simulink model "LBSSHA005_EEE4119F_Project"  (R2021a)
settings: Solver=VariableStepAuto  StartTime=0.0  StopTime=60  RelTol=1e-3
undefined symbols (not defined in the file or in its folder): Klqr, Klqr_b, Kr, Kr_b
libraries: dspsigops x1
settings Model: EnablePacing=on  Creator=Administrator  LastModifiedBy=shaun
settings SolverCC: ZeroCrossAlgorithm=Adaptive
settings DebuggingCC: IgnoredZcDiagnostic=none

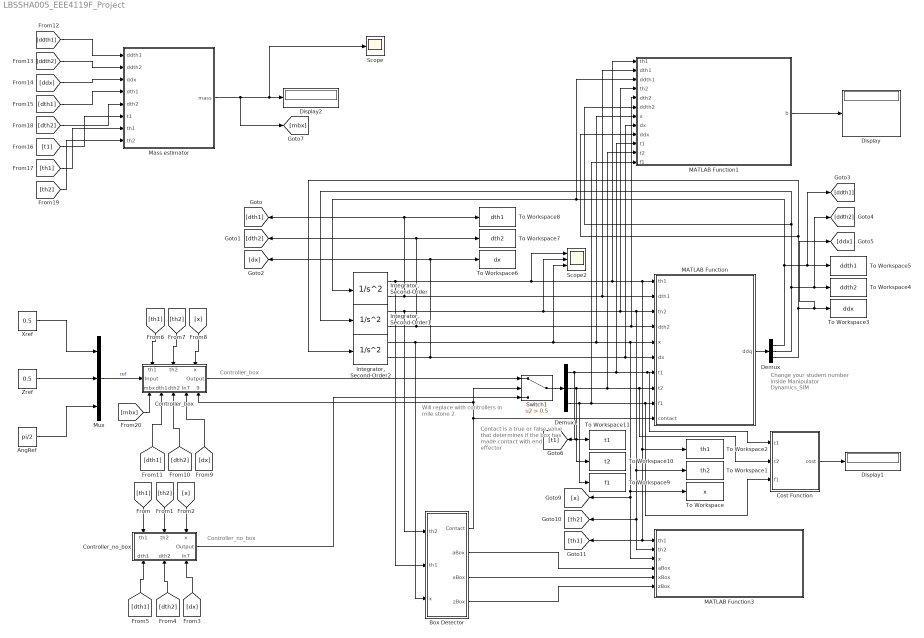
== system LBSSHA005_EEE4119F_Project ==
  note: Controller_box
  note: Controller_no_box
  note: Contact is a true or false value that determines if the box has made contact with end effector
  note: Will replace with controllers in mile stone 2
  note: Change your student number inside Manipulator Dynamics_SIM
  AngRef : Constant  Value=pi/2
  Box Detector : Subsystem
  Controller_box : Subsystem
      settings: PortSchema="{\"entries\":[{\"content\":{\"sides\":[{\"content\":{\"connectorIds\":[\"In1\"]},\"type\":\"ConnectorPlacement.EquallySpacedRectSide\",\"uuid\":\"442c6cb1-0c83-47f7-ad07-2f020ac45e6e\"},{\"content\":{\"connectorIds\":[\"Out1\"],\"side\":\"RIGHT\"},\"type\":\"ConnectorPlacement.EquallySpacedRectSide\",\"uuid\":\"7f993a2f-adf1-4607-9f11-cdbb59b13442\"},{\"content\":{\"connectorIds\":[\"In2\",\"In3\",\"In4\"],\"side\":\"TOP\"},\"type\":\"ConnectorPlacement.EquallySpacedRectSide\",\"uuid\":\"5e67f2e7-af9c-4bde-80a5-b1ef30d10dbb\"},{\"content\":{\"connectorIds\":[\"In5\",\"In6\",\"In7\",\"In8\",\"In9\"],\"side\":\"BOTTOM\"},\"type\":\"ConnectorPlacement.EquallySpacedRectSide\",\"uuid\":\"20da8873-f5b9-43e3-93ec-958325ed584f\"}]},\"type\":\"ConnectorPlacement.EquallySpacedConnector\",\"uuid\":\"88c068a2-7487-43c4-b188-48c79a1dd5d7\"}],\"packageUris\":[\"http://schema.mathworks.com/mf0/Connector/R2020b\"],\"version\":\"1.0\"}"
  Controller_no_box : Subsystem
      settings: PortSchema="{\"entries\":[{\"content\":{\"sides\":[{\"content\":{\"connectorIds\":[]},\"type\":\"ConnectorPlacement.EquallySpacedRectSide\",\"uuid\":\"88738e74-d91b-4dc7-a725-58f175a94349\"},{\"content\":{\"connectorIds\":[\"Out1\"],\"side\":\"RIGHT\"},\"type\":\"ConnectorPlacement.EquallySpacedRectSide\",\"uuid\":\"6cf3a578-d327-404a-bf63-fc00ab4a30ba\"},{\"content\":{\"connectorIds\":[\"In1\",\"In2\",\"In3\"],\"side\":\"TOP\"},\"type\":\"ConnectorPlacement.EquallySpacedRectSide\",\"uuid\":\"b92cd528-6e23-44bd-9603-b71daa2ffdae\"},{\"content\":{\"connectorIds\":[\"In4\",\"In5\",\"In6\"],\"side\":\"BOTTOM\"},\"type\":\"ConnectorPlacement.EquallySpacedRectSide\",\"uuid\":\"f1bd1ac8-fd96-4684-af34-69bf2dd321d9\"}]},\"type\":\"ConnectorPlacement.EquallySpacedConnector\",\"uuid\":\"af1ac5a9-5139-4c84-9774-81cc3394ecc5\"}],\"packageUris\":[\"http://schema.mathworks.com/mf0/Connector/R2020b\"],\"version\":\"1.0\"}"
  Cost Function : Subsystem
  Demux : Demux  Outputs=3
  Demux1 : Demux  Outputs=3
  Display : Display
  Display1 : Display
  Display2 : Display
  "Integrator, Second-Order" : SecondOrderIntegrator
  "Integrator, Second-Order1" : SecondOrderIntegrator  ICX=0
  "Integrator, Second-Order2" : SecondOrderIntegrator  ICX=0
  MATLAB Function : MATLAB Function  TreatAsAtomicUnit=on
  MATLAB Function1 : MATLAB Function  TreatAsAtomicUnit=on
  MATLAB Function3 : MATLAB Function  TreatAsAtomicUnit=on  SystemSampleTime=0.15
  Mass estimator : MATLAB Function  TreatAsAtomicUnit=on
  Mux : Mux  Inputs=3
  Scope : Scope
  Scope2 : Scope  NumInputPorts=3
  Switch1 : Switch  Criteria=u2 > Threshold  Threshold=0.5
  To Workspace : ToWorkspace  VariableName=x  SaveFormat=Structure With Time  SampleTime=-1
  To Workspace1 : ToWorkspace  VariableName=th2  SaveFormat=Structure With Time  SampleTime=-1
  To Workspace10 : ToWorkspace  VariableName=t2  SaveFormat=Structure With Time  SampleTime=-1
  To Workspace11 : ToWorkspace  VariableName=t1  SaveFormat=Structure With Time  SampleTime=-1
  To Workspace2 : ToWorkspace  VariableName=th1  SaveFormat=Structure With Time  SampleTime=-1
  To Workspace3 : ToWorkspace  VariableName=ddx  SaveFormat=Structure With Time  SampleTime=-1
  To Workspace4 : ToWorkspace  VariableName=ddth2  SaveFormat=Structure With Time  SampleTime=-1
  To Workspace5 : ToWorkspace  VariableName=ddth1  SaveFormat=Structure With Time  SampleTime=-1
  To Workspace6 : ToWorkspace  VariableName=dx  SaveFormat=Structure With Time  SampleTime=-1
  To Workspace7 : ToWorkspace  VariableName=dth2  SaveFormat=Structure With Time  SampleTime=-1
  To Workspace8 : ToWorkspace  VariableName=dth1  SaveFormat=Structure With Time  SampleTime=-1
  To Workspace9 : ToWorkspace  VariableName=f1  SaveFormat=Structure With Time  SampleTime=-1
  Xref : Constant  Value=0.5
  Zref : Constant  Value=0.5
  wires:
  Demux/1 -> [ddth1], To Workspace5/1, MATLAB Function1/3(ddth1), "Integrator, Second-Order"/1
  Demux/2 -> [ddth2], To Workspace4/1, MATLAB Function1/6(ddth2), "Integrator, Second-Order1"/1
  MATLAB Function/1(ddq) -> Demux/1
  "Integrator, Second-Order1"/2 -> [dth2], To Workspace7/1, MATLAB Function1/5(dth2), MATLAB Function/4(dth2)
  Demux1/1 -> [t1], To Workspace11/1, MATLAB Function1/10(t1), Cost Function/1(t1), MATLAB Function/7(t1)
  "Integrator, Second-Order"/1 -> Box Detector/2(th1), Scope2/1, MATLAB Function1/1(th1), MATLAB Function3/1(th1), [th1], To Workspace2/1, MATLAB Function/1(th1)
  "Integrator, Second-Order1"/1 -> Box Detector/1(th2), [th2], MATLAB Function3/2(th2), To Workspace1/1, MATLAB Function/3(th2), MATLAB Function1/4(th2), Scope2/2
  "Integrator, Second-Order2"/2 -> [dx], To Workspace6/1, MATLAB Function1/8(dx), MATLAB Function/6(dx)
  Demux/3 -> [ddx], To Workspace3/1, MATLAB Function1/9(ddx), "Integrator, Second-Order2"/1
  "Integrator, Second-Order2"/1 -> Scope2/3, MATLAB Function1/7(x), [x], MATLAB Function3/3(x), To Workspace/1, MATLAB Function/5(x), Box Detector/3(x)
  "Integrator, Second-Order"/2 -> To Workspace8/1, [dth1], MATLAB Function1/2(dth1), MATLAB Function/2(dth1)
  Demux1/2 -> To Workspace10/1, Cost Function/2(t2), MATLAB Function/8(t2), MATLAB Function1/11(t2)
  Demux1/3 -> To Workspace9/1, Cost Function/3(f1), MATLAB Function/9(f1), MATLAB Function1/12(f1)
  Switch1/1 -> Demux1/1
  Box Detector/4(zBox) -> MATLAB Function3/6(zBox)
  Box Detector/3(xBox) -> MATLAB Function3/5(xBox)
  Box Detector/2(aBox) -> MATLAB Function3/4(aBox)
  Box Detector/1(Contact) -> Controller_box/9(Contact), Switch1/2, MATLAB Function/10(contact)
  MATLAB Function1/1(b) -> Display/1
  [th1] -> Controller_no_box/1(th1)
  [th2] -> Controller_no_box/2(th2)
  [x] -> Controller_no_box/3(x)
  [dth1] -> Controller_no_box/4(dth1)
  [dth2] -> Controller_no_box/5(dth2)
  [dx] -> Controller_no_box/6(In7)
  [th2] -> Controller_box/3(th2)
  [th1] -> Controller_box/2(th1)
  [x] -> Controller_box/4(x)
  [dx] -> Controller_box/8(In7)
  [dth2] -> Controller_box/7(dth2)
  [dth1] -> Controller_box/6(dth1)
  Controller_box/1(Output) -> Switch1/1
  Controller_no_box/1(Output) -> Switch1/3
  Zref/1 -> Mux/2
  Xref/1 -> Mux/1
  AngRef/1 -> Mux/3
  Mux/1 -> Controller_box/1(Input)  "ref"
  Cost Function/1(cost) -> Display1/1
  [ddth1] -> Mass estimator/1(ddth1)
  [ddth2] -> Mass estimator/2(ddth2)
  [ddx] -> Mass estimator/3(ddx)
  [dth1] -> Mass estimator/4(dth1)
  [dth2] -> Mass estimator/5(dth2)
  [t1] -> Mass estimator/6(t1)
  [th1] -> Mass estimator/7(th1)
  [th2] -> Mass estimator/8(th2)
  Mass estimator/1(mass) -> [mbx], Scope/1, Display2/1
  [mbx] -> Controller_box/5(mbx)

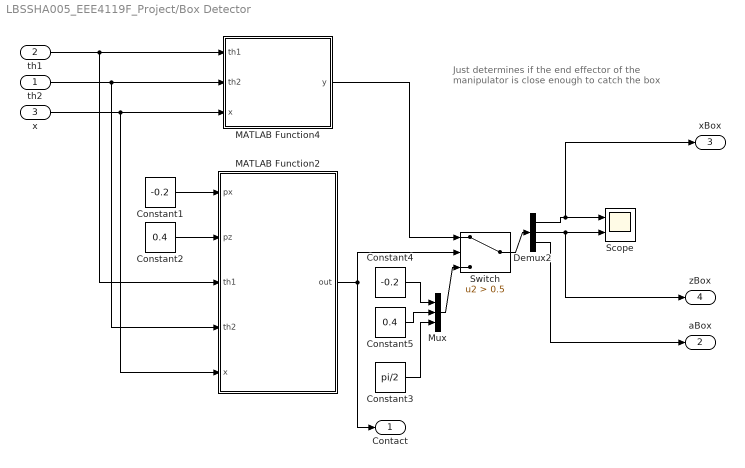
== system LBSSHA005_EEE4119F_Project/Box Detector ==
  note: Just determines if the end effector of the manipulator is close enough to catch the box
  th2 : Inport
  th1 : Inport  Port=2
  x : Inport  Port=3
  Constant1 : Constant  Value=-0.2
  Constant2 : Constant  Value=0.4
  Constant3 : Constant  Value=pi/2
  Constant4 : Constant  Value=-0.2
  Constant5 : Constant  Value=0.4
  Demux2 : Demux  Outputs=3
  MATLAB Function2 : MATLAB Function  TreatAsAtomicUnit=on
  MATLAB Function4 : MATLAB Function  TreatAsAtomicUnit=on
  Mux : Mux  Inputs=3
  Scope : Scope  NumInputPorts=2
  Switch : Switch  Criteria=u2 > Threshold  Threshold=0.5
  Contact : Outport
  aBox : Outport  Port=2
  xBox : Outport  Port=3
  zBox : Outport  Port=4
  wires:
  Demux2/2 -> zBox/1, Scope/2
  Mux/1 -> Switch/3
  Constant5/1 -> Mux/2
  MATLAB Function4/1(y) -> Switch/1
  Demux2/1 -> Scope/1, xBox/1
  Constant4/1 -> Mux/1
  Switch/1 -> Demux2/1
  x/1 -> MATLAB Function2/5(x), MATLAB Function4/3(x)
  th1/1 -> MATLAB Function2/3(th1), MATLAB Function4/1(th1)
  th2/1 -> MATLAB Function2/4(th2), MATLAB Function4/2(th2)
  MATLAB Function2/1(out) -> Switch/2, Contact/1
  Constant1/1 -> MATLAB Function2/1(px)
  Constant2/1 -> MATLAB Function2/2(pz)
  Demux2/3 -> aBox/1
  Constant3/1 -> Mux/3

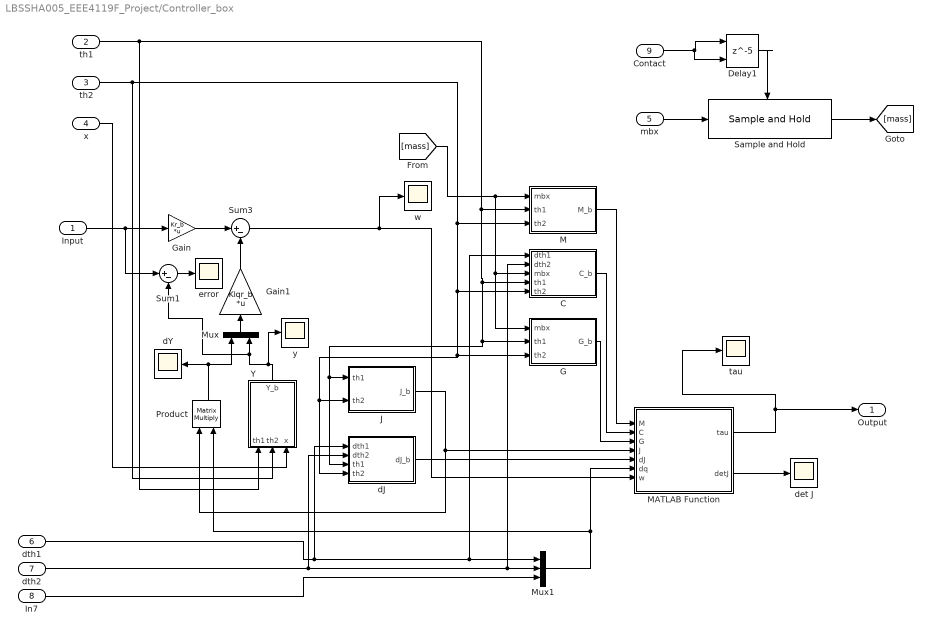
== system LBSSHA005_EEE4119F_Project/Controller_box ==
  Input : Inport
  th1 : Inport  Port=2
  th2 : Inport  Port=3
  x : Inport  Port=4
  mbx : Inport  Port=5
  dth1 : Inport  Port=6
  dth2 : Inport  Port=7
  In7 : Inport  Port=8
  Contact : Inport  Port=9
  C : MATLAB Function  TreatAsAtomicUnit=on
  Delay1 : Delay  DelayLength=5  ExternalReset=Rising
      settings: InputPortMap=u0,r5
  G : MATLAB Function  TreatAsAtomicUnit=on
  Gain : Gain  Gain=Kr_b  Multiplication=Matrix(K*u)
  Gain1 : Gain  Gain=Klqr_b  Multiplication=Matrix(K*u)
  J : MATLAB Function  TreatAsAtomicUnit=on
  M : MATLAB Function  TreatAsAtomicUnit=on
  MATLAB Function : MATLAB Function  TreatAsAtomicUnit=on
  Mux : Mux  Inputs=2
  Mux1 : Mux  Inputs=3
  Product : Product  Multiplication=Matrix(*)
  Sample and Hold : dspsigops/Sample and Hold  trig=Rising edge  initCond=1  latchinput=on
  Sum1 : Sum  Inputs=|+-
  Sum3 : Sum  Inputs=|+-
  Y : MATLAB Function  TreatAsAtomicUnit=on
  dJ : MATLAB Function  TreatAsAtomicUnit=on
  dY : Scope
  det J : Scope
  error : Scope
  tau : Scope
  w : Scope
  y : Scope
  Output : Outport
  wires:
  J/1(J_b) -> MATLAB Function/4(J), Product/1
  Gain1/1 -> Sum3/2
  Y/1(Y_b) -> Sum1/2, Mux/2, y/1
  Product/1 -> dY/1, Mux/1
  MATLAB Function/1(tau) -> Output/1, tau/1
  Mux/1 -> Gain1/1
  dJ/1(dJ_b) -> MATLAB Function/5(dJ)
  Sum3/1 -> MATLAB Function/7(w), w/1
  Input/1 -> Gain/1, Sum1/1
  MATLAB Function/2(detJ) -> det J/1
  Sum1/1 -> error/1
  M/1(M_b) -> MATLAB Function/1(M)
  C/1(C_b) -> MATLAB Function/2(C)
  G/1(G_b) -> MATLAB Function/3(G)
  th1/1 -> Y/1(th1), G/2(th1), dJ/3(th1), J/1(th1), C/4(th1), M/2(th1)
  th2/1 -> Y/2(th2), G/3(th2), dJ/4(th2), J/2(th2), C/5(th2), M/3(th2)
  x/1 -> Y/3(x)
  dth1/1 -> C/1(dth1), Mux1/1, dJ/1(dth1)
  dth2/1 -> C/2(dth2), Mux1/2, dJ/2(dth2)
  In7/1 -> Mux1/3
  Mux1/1 -> MATLAB Function/6(dq), Product/2
  Gain/1 -> Sum3/1
  Delay1/1 -> Sample and Hold/Trigger
  Sample and Hold/1 -> [mass]
  [mass] -> M/1(mbx), G/1(mbx), C/3(mbx)
  mbx/1 -> Sample and Hold/1
  Contact/1 -> Delay1/2, Delay1/1

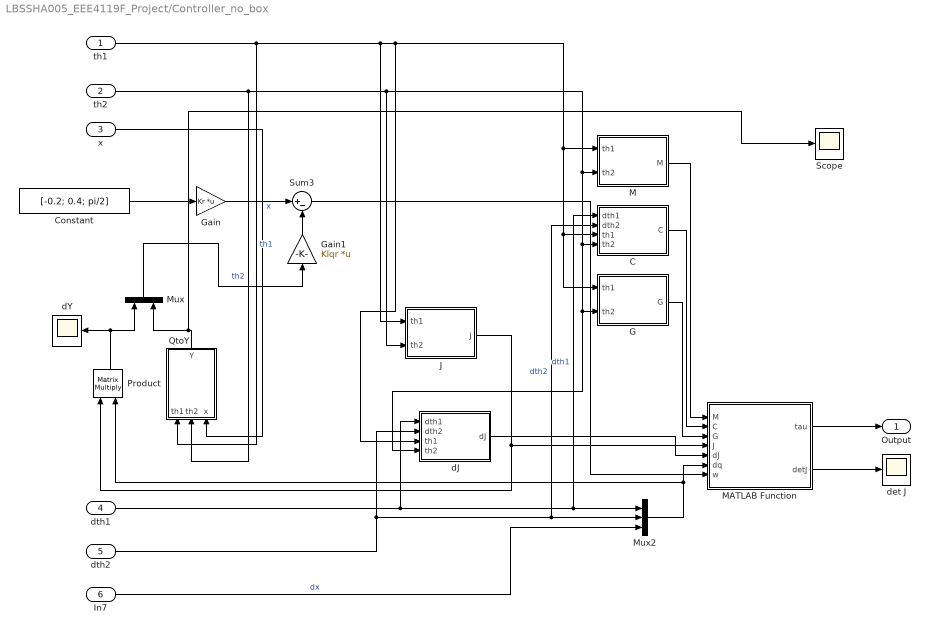
== system LBSSHA005_EEE4119F_Project/Controller_no_box ==
  th1 : Inport
  th2 : Inport  Port=2
  x : Inport  Port=3
  dth1 : Inport  Port=4
  dth2 : Inport  Port=5
  In7 : Inport  Port=6
  C : MATLAB Function  TreatAsAtomicUnit=on
  Constant : Constant  Value=[-0.2; 0.4; pi/2]
  G : MATLAB Function  TreatAsAtomicUnit=on
  Gain : Gain  Gain=Kr  Multiplication=Matrix(K*u)
  Gain1 : Gain  Gain=Klqr  Multiplication=Matrix(K*u)
  J : MATLAB Function  TreatAsAtomicUnit=on
  M : MATLAB Function  TreatAsAtomicUnit=on
  MATLAB Function : MATLAB Function  TreatAsAtomicUnit=on
  Mux : Mux  Inputs=2
  Mux2 : Mux  Inputs=3
  Product : Product  Multiplication=Matrix(*)
  QtoY : MATLAB Function  TreatAsAtomicUnit=on
  Scope : Scope
  Sum3 : Sum  Inputs=|+-
  dJ : MATLAB Function  TreatAsAtomicUnit=on
  dY : Scope
  det J : Scope
  Output : Outport
  wires:
  M/1(M) -> MATLAB Function/1(M)
  J/1(J) -> MATLAB Function/4(J), Product/1
  Gain1/1 -> Sum3/2
  QtoY/1(Y) -> Scope/1, Mux/2
  Product/1 -> dY/1, Mux/1
  MATLAB Function/1(tau) -> Output/1
  Mux/1 -> Gain1/1
  dJ/1(dJ) -> MATLAB Function/5(dJ)
  Sum3/1 -> MATLAB Function/7(w)
  Constant/1 -> Gain/1
  C/1(C) -> MATLAB Function/2(C)
  MATLAB Function/2(detJ) -> det J/1
  dth1/1 -> C/1(dth1), Mux2/1, dJ/1(dth1)  "dth1"
  dth2/1 -> C/2(dth2), Mux2/2, dJ/2(dth2)  "dth2"
  In7/1 -> Mux2/3  "dx"
  Mux2/1 -> MATLAB Function/6(dq), Product/2
  th2/1 -> J/2(th2), C/4(th2), dJ/4(th2), G/2(th2), M/2(th2), QtoY/2(th2)  "th2"
  x/1 -> QtoY/3(x)  "x"
  th1/1 -> dJ/3(th1), C/3(th1), G/1(th1), M/1(th1), J/1(th1), QtoY/1(th1)  "th1"
  G/1(G) -> MATLAB Function/3(G)
  Gain/1 -> Sum3/1

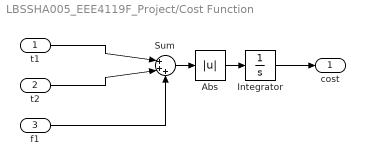
== system LBSSHA005_EEE4119F_Project/Cost Function ==
  t1 : Inport
  t2 : Inport  Port=2
  f1 : Inport  Port=3
  Abs : Abs
  Integrator : Integrator
  Sum : Sum  Inputs=|+++
  cost : Outport
  wires:
  Sum/1 -> Abs/1
  f1/1 -> Sum/3
  t2/1 -> Sum/2
  Integrator/1 -> cost/1
  t1/1 -> Sum/1
  Abs/1 -> Integrator/1

== matlab function LBSSHA005_EEE4119F_Project/Controller_no_box/C ==
  data: C output; dth1 input; dth2 input; th1 input; th2 input
function C = C(dth1,dth2,th1,th2)
%#codegen

%    This function was generated by the Symbolic Math Toolbox version 8.7.
%    13-May-2022 16:47:02

t2 = sin(th2);
t3 = th1+th2;
t4 = cos(t3);
C = [dth2.*t2.*(dth1.*2.0+dth2).*(-1.0./1.28e+2);(dth1.^2.*t2)./1.28e+2;-dth1.*(dth1.*(t4./3.2e+1+cos(th1).*(3.0./3.2e+1))+(dth2.*t4)./3.2e+1)-(dth2.*t4.*(dth1+dth2))./3.2e+1];

== matlab function LBSSHA005_EEE4119F_Project/Controller_no_box/QtoY ==
  data: th1 input; Y output; th2 input; x input
function Y = QtoY(th1,th2,x)
%#codegen

%    This function was generated by the Symbolic Math Toolbox version 8.7.
%    13-May-2022 16:47:02

t2 = cos(th1);
t3 = cos(th2);
t4 = sin(th1);
t5 = sin(th2);
Y = [t2./4.0+x+(t2.*t3)./4.0-(t4.*t5)./4.0;t4./4.0+(t2.*t5)./4.0+(t3.*t4)./4.0;th1+th2];

== matlab function LBSSHA005_EEE4119F_Project/Controller_box/MATLAB Function ==
  data: M input; tau output; C input; G input; J input; dJ input; dq input; w input; detJ output
function [tau,detJ] = fcn(M, C, G, J, dJ, dq, w)

% Mapping the nonlinear control - used Jacobian Transpose Method
% (https://journals.sagepub.com/doi/pdf/10.1177/0278364917698748)
% J\ - could try this...
% pinv(J) - could also try this...
% Check that Jaocbian is not singular. If singular rather use transpose.
b = 0.8353;
G = transpose(G);
if abs(det(J)) < 1e-3
    tau = M*(J'*(w-dJ*dq)) + C + G + b*dq;
else
    tau = M*(J\(w-dJ*dq)) + C + G + b*dq;
end

detJ = det(J);
% see http://www.cs.columbia.edu/~allen/F15/NOTES/jacobians.pdf for further
% clarity on Jacobians going singular. Short answer: this happens when a robot loses a degree
% of freedom, similar to what we discussed in class about Gimbal Lock

== matlab function LBSSHA005_EEE4119F_Project/Controller_no_box/dJ ==
  data: dth1 input; dJ output; dth2 input; th1 input; th2 input
function dJ = dJ(dth1,dth2,th1,th2)
%#codegen

%    This function was generated by the Symbolic Math Toolbox version 8.7.
%    13-May-2022 16:47:03

t2 = th1+th2;
t3 = cos(t2);
t4 = sin(t2);
t5 = (dth2.*t3)./4.0;
t6 = (dth2.*t4)./4.0;
t7 = -t5;
t8 = -t6;
dJ = reshape([t7-(dth1.*(t3+cos(th1)))./4.0,t8-(dth1.*(t4+sin(th1)))./4.0,0.0,t7-(dth1.*t3)./4.0,t8-(dth1.*t4)./4.0,0.0,0.0,0.0,0.0],[3,3]);

== matlab function LBSSHA005_EEE4119F_Project/Controller_box/M ==
  data: mbx input; th1 input; M_b output; th2 input
function M_b = M(mbx,th1,th2)
%#codegen

%    This function was generated by the Symbolic Math Toolbox version 8.7.
%    13-May-2022 16:47:03

t2 = cos(th1);
t3 = sin(th1);
t4 = th1+th2;
t13 = mbx./3.0e+2;
t5 = cos(t4);
t6 = sin(t4);
t9 = t2./4.0;
t10 = t3./2.0;
t11 = t3./4.0;
t12 = t3.*(3.0./3.2e+1);
t7 = t5.^2;
t8 = t6.^2;
t14 = t6.*(3.0./5.0);
t15 = -t12;
t16 = t5./8.0;
t17 = t5.*(3.0./1.0e+1);
t18 = t6./8.0;
t19 = t6.*(3.0./1.0e+1);
t20 = t6./3.2e+1;
t23 = mbx.*t6.*(-3.0./1.0e+1);
t21 = -t20;
t22 = mbx.*t19;
t24 = t10+t14;
t25 = t9+t16;
t26 = t9+t17;
t27 = t11+t18;
t28 = t11+t19;
t29 = (mbx.*t24)./2.0;
t31 = t21+t23;
t32 = (t5.*t25)./3.2e+1;
t33 = t20.*t27;
t34 = mbx.*t17.*t26;
t35 = t22.*t28;
t30 = -t29;
t37 = t13+t32+t33+t34+t35+1.0./1.92e+2;
t36 = t15+t21+t30;
M_b = reshape([t13+cos(th1.*2.0)./5.12e+2+mbx.*t26.^2+mbx.*t28.^2+t3.^2./2.56e+2+t25.^2./4.0+t27.^2./4.0+1.236979166666667e-2,t37,t36,t37,t7./2.56e+2+t8./2.56e+2+t13+mbx.*t7.*(9.0./1.0e+2)+mbx.*t8.*(9.0./1.0e+2)+1.0./1.92e+2,t31,t36,t31,mbx+3.0./4.0],[3,3]);

== matlab function LBSSHA005_EEE4119F_Project/Controller_box/G ==
  data: mbx input; th1 input; G_b output; th2 input
function G_b = G(mbx,th1,th2)
%#codegen

%    This function was generated by the Symbolic Math Toolbox version 8.7.
%    13-May-2022 16:47:04

t2 = cos(th1);
t3 = th1+th2;
t4 = cos(t3);
G_b = [t2.*9.196875e-1+t4.*3.065625e-1+mbx.*(t2./4.0+t4.*(3.0./1.0e+1)).*(9.81e+2./1.0e+2),t4.*(mbx.*(3.0./5.0)+1.0./1.6e+1).*(9.81e+2./2.0e+2),0.0];

== matlab function LBSSHA005_EEE4119F_Project/Controller_box/C ==
  data: dth1 input; C_b output; dth2 input; mbx input; th1 input; th2 input
function C_b = C(dth1,dth2,mbx,th1,th2)
%#codegen

%    This function was generated by the Symbolic Math Toolbox version 8.7.
%    13-May-2022 16:47:04

t2 = cos(th1);
t3 = sin(th2);
t4 = th1+th2;
t6 = mbx.*(3.0./5.0);
t5 = cos(t4);
t8 = t6+1.0./1.6e+1;
t7 = t5./3.2e+1;
C_b = [dth2.*t3.*t8.*(dth1.*2.0+dth2).*(-1.0./8.0);(dth1.^2.*t3.*t8)./8.0;-dth1.*(dth1.*(t2.*(3.0./3.2e+1)+t7+(mbx.*(t2./2.0+t5.*(3.0./5.0)))./2.0)+dth2.*(t7+mbx.*t5.*(3.0./1.0e+1)))-(dth2.*t5.*t8.*(dth1+dth2))./2.0];

== matlab function LBSSHA005_EEE4119F_Project/Controller_box/J ==
  data: th1 input; J_b output; th2 input
function J_b = J(th1,th2)
%#codegen

%    This function was generated by the Symbolic Math Toolbox version 8.7.
%    13-May-2022 16:47:05

t2 = th1+th2;
t3 = cos(t2);
t4 = sin(t2);
t5 = t3.*(3.0./1.0e+1);
t6 = t4.*(3.0./1.0e+1);
t7 = -t6;
J_b = reshape([t7-sin(th1)./4.0,t5+cos(th1)./4.0,1.0,t7,t5,1.0,1.0,0.0,0.0],[3,3]);

== matlab function LBSSHA005_EEE4119F_Project/MATLAB Function1 ==
  data: th1 input; b output; dth1 input; ddth1 input; th2 input; dth2 input; ddth2 input; x input; dx input; ddx input; t1 input; t2 input; f1 input
function b = extractb(th1, dth1, ddth1,th2, dth2, ddth2, x, dx, ddx,t1, t2, f1)

m = 0.25;
L = 0.25;
g = 9.81;
Jyy = (1/3)*m*L^2;
dq = [dth1;dth2;dx];
t = [t1;t2;f1];
ddq = [ddth1;ddth2;ddx];

M = [2*Jyy + (3*L^2*m)/2 + L^2*m*cos(th2), Jyy + (L^2*m)/4 + (L^2*m*cos(th2))/2, - (3*L*m*sin(th1))/2 - (L*m*sin(th1 + th2))/2; Jyy + (L^2*m)/4 + (L^2*m*cos(th2))/2, (m*L^2)/4 + Jyy, -(L*m*sin(th1 + th2))/2; - (3*L*m*sin(th1))/2 - (L*m*sin(th1 + th2))/2, -(L*m*sin(th1 + th2))/2, 3*m];

G = [(L*g*m*(cos(th1 + th2) + 3*cos(th1)))/2, (L*g*m*cos(th1 + th2))/2, 0];

C = [-(L^2*dth2*m*sin(th2)*(2*dth1 + dth2))/2; (L^2*dth1^2*m*sin(th2))/2; - dth1*(dth1*((L*m*cos(th1 + th2))/2 + (3*L*m*cos(th1))/2) + (L*dth2*m*cos(th1 + th2))/2) - (L*dth2*m*cos(th1 + th2)*(dth1 + dth2))/2];

A = diag(dq);
B = -(M*ddq + C + transpose(G) - t);
b = A\B;

== matlab function LBSSHA005_EEE4119F_Project/Controller_box/dJ ==
  data: dth1 input; dJ_b output; dth2 input; th1 input; th2 input
function dJ_b = dJ(dth1,dth2,th1,th2)
%#codegen

%    This function was generated by the Symbolic Math Toolbox version 8.7.
%    13-May-2022 16:47:05

t2 = th1+th2;
t3 = cos(t2);
t4 = sin(t2);
t5 = dth2.*t3.*(3.0./1.0e+1);
t6 = dth2.*t4.*(3.0./1.0e+1);
t7 = -t5;
t8 = -t6;
dJ_b = reshape([t7-dth1.*(t3.*(3.0./1.0e+1)+cos(th1)./4.0),t8-dth1.*(t4.*(3.0./1.0e+1)+sin(th1)./4.0),0.0,t7-dth1.*t3.*(3.0./1.0e+1),t8-dth1.*t4.*(3.0./1.0e+1),0.0,0.0,0.0,0.0],[3,3]);

== matlab function LBSSHA005_EEE4119F_Project/Controller_box/Y ==
  data: th1 input; Y_b output; th2 input; x input
function Y_b = Y(th1,th2,x)
%#codegen

%    This function was generated by the Symbolic Math Toolbox version 8.7.
%    13-May-2022 16:47:05

t2 = cos(th1);
t3 = cos(th2);
t4 = sin(th1);
t5 = sin(th2);
Y_b = [t2./4.0+x+t2.*t3.*(3.0./1.0e+1)-t4.*t5.*(3.0./1.0e+1);t4./4.0+t2.*t5.*(3.0./1.0e+1)+t3.*t4.*(3.0./1.0e+1);th1+th2];

== matlab function LBSSHA005_EEE4119F_Project/Mass estimator ==
  data: ddth1 input; mass output; ddth2 input; ddx input; dth1 input; dth2 input; t1 input; th1 input; th2 input
function mass = MassEstimator(ddth1,ddth2,ddx,dth1,dth2,t1,th1,th2)
%#codegen

%    This function was generated by the Symbolic Math Toolbox version 8.7.
%    13-May-2022 16:37:49

t3 = cos(th1);
t4 = sin(th1);
t5 = sin(th2);
t6 = th1+th2;
t7 = dth1.*2.0;
t8 = cos(t6);
t9 = sin(t6);
t10 = dth2+t7;
t11 = t3./4.0;
t12 = t4./4.0;
t13 = t8./8.0;
t14 = t8.*(3.0./1.0e+1);
t15 = t9./8.0;
t16 = t9.*(3.0./1.0e+1);
t17 = t11+t13;
t18 = t11+t14;
t19 = t12+t15;
t20 = t12+t16;
et1 = (-t1+t3.*9.196875e-1+t8.*3.065625e-1+th1.*8.353e-1+ddth1.*(cos(th1.*2.0)./5.12e+2+t4.^2./2.56e+2+t17.^2./4.0+t19.^2./4.0+1.236979166666667e-2)+ddth2.*((t8.*t17)./3.2e+1+(t9.*t19)./3.2e+1+1.0./1.92e+2)-ddx.*(t4.*(3.0./3.2e+1)+t9./3.2e+1)-(dth2.*t5.*t10)./1.28e+2)./(t3.*(9.81e+2./4.0e+2)+t8.*2.943-ddx.*t20+ddth2.*(t14.*t18+t16.*t20+1.0./3.0e+2)+ddth1.*(t18.^2+t20.^2+1.0./3.0e+2)-dth2.*t5.*t10.*(3.0./4.0e+1));
et2 = -1.0;
mass = et1.*et2;

== matlab function LBSSHA005_EEE4119F_Project/Controller_no_box/MATLAB Function ==
  data: M input; tau output; C input; G input; J input; dJ input; dq input; w input; detJ output
function [tau,detJ] = fcn(M, C, G, J, dJ, dq, w)

% Mapping the nonlinear control - used Jacobian Transpose Method
% (https://journals.sagepub.com/doi/pdf/10.1177/0278364917698748)
% J\ - could try this...
% pinv(J) - could also try this...
% Check that Jaocbian is not singular. If singular rather use transpose.
b = 0.8353;
G = transpose(G);
if abs(det(J)) < 1e-3
    tau = M*(J'*(w-dJ*dq)) + C + G + b*dq;
else
    tau = M*(J\(w-dJ*dq)) + C + G + b*dq;
end

detJ = det(J);
% see http://www.cs.columbia.edu/~allen/F15/NOTES/jacobians.pdf for further
% clarity on Jacobians going singular. Short answer: this happens when a robot loses a degree
% of freedom, similar to what we discussed in class about Gimbal Lock

== matlab function LBSSHA005_EEE4119F_Project/MATLAB Function ==
  data: th1 input; dth1 input; th2 input; dth2 input; x input; dx input; ddq output; t1 input; t2 input; f1 input; contact input
function ddq = ManipulatorDynamics_SIM(th1, dth1,th2, dth2,x, dx, t1, t2, f1, contact)
    coder.extrinsic('ManipulatorDynamics');
    STDNUM = 'LBSSHA005';
    
    % I will give you this function later when we deal with unknown loads 
    coder.extrinsic('BoxMass');
    boxMass = BoxMass('LBSSHA005',2);
    % boxMass = 1;
  
    ddq = [0;0;0];
    ddq = ManipulatorDynamics(th1, dth1,th2, dth2,x, dx, t1, t2, f1, contact, STDNUM, boxMass);
end

== matlab function LBSSHA005_EEE4119F_Project/Box Detector/MATLAB Function2 ==
  settings: updateMethod=DISCRETE
  data: px input; out output; pz input; th1 input; th2 input; x input
function out  = Object_Sensor(px,pz,th1,th2,x)
persistent flag
if isempty(flag)
    flag = 0;
end
y = [x+0.25*cos(th1)+0.25*cos(th1+th2);...
         0.25*sin(th1)+0.25*sin(th1+th2);...
         th1+th2];
target = [px;pz;pi/2];
e = target-y;
epsilon = 0.001;
if (e(1) <= epsilon) && (e(2) <= epsilon) && (e(3)<= epsilon)
    out = 1;
    flag = 1;
else
    out = 0;
end
if flag == 1
    out =1;
end 
end

== matlab function LBSSHA005_EEE4119F_Project/Controller_no_box/M ==
  data: th1 input; M output; th2 input
function M = M(th1,th2)
%#codegen

%    This function was generated by the Symbolic Math Toolbox version 8.7.
%    13-May-2022 16:47:01

t2 = cos(th2);
t3 = sin(th1);
t4 = th1+th2;
t5 = sin(t4);
t6 = t3.*(3.0./3.2e+1);
t7 = t2./1.28e+2;
t8 = -t6;
t9 = t5./3.2e+1;
t11 = t7+7.0./7.68e+2;
t10 = -t9;
t12 = t8+t10;
M = reshape([t2./6.4e+1+1.3e+1./3.84e+2,t11,t12,t11,7.0./7.68e+2,t10,t12,t10,3.0./4.0],[3,3]);

== matlab function LBSSHA005_EEE4119F_Project/Box Detector/MATLAB Function4 ==
  data: th1 input; y output; th2 input; x input
function y = endEffector(th1,th2,x)
y = [x + 0.25*cos(th1)+0.25*cos(th1+th2);...
     0.25*sin(th1)+0.25*sin(th1+th2);...
     th1+th2];
end

== matlab function LBSSHA005_EEE4119F_Project/MATLAB Function3 ==
  settings: updateMethod=DISCRETE
  data: th1 input; th2 input; x input; aBox input; xBox input; zBox input
function Animate(th1, th2, x, aBox, xBox, zBox)
coder.extrinsic('patch'); 
coder.extrinsic('GeoVerMakeCyl'); 
coder.extrinsic('GeoVerMakeBlock'); 
coder.extrinsic('GeoPatMakeCyl'); 
coder.extrinsic('GeoPatMakeBlock'); 
Base_x = 0.15;
Base_y = 0.15;
Base_z = 0.15;
L = 0.25;

blockColour = 'c';
% you don't really need to understand the code below

%% Draw rail
% Calculate Rotation Matrix - from inertial to body
% Compute propagation of vertices and patches
temp = [-0.59, 0.075, -0.15/2+0.075];
Vertex5Data = GeoVerMakeBlock(temp, eye(3), [2*0.59,Base_y/4,Base_z/4]);
[X,Y,Z] = GeoPatMakeBlock(Vertex5Data);
    
Patch5Data_X = X;
Patch5Data_Y = Y;
Patch5Data_Z = Z;

%% Draw Base
% Calculate Rotation Matrix - from inertial to body
% Compute propagation of vertices and patches
temp = [x-0.15/2, 0.025, -0.15/2];
VertexData = GeoVerMakeBlock(temp, eye(3), [Base_x,Base_y,Base_z]);
[X,Y,Z] = GeoPatMakeBlock(VertexData);
   
PatchData_X = X;
PatchData_Y = Y;
PatchData_Z = Z;
%% Draw Link 1
% Calculate Rotation Matrix - from inertial to body
% Compute propagation of vertices and patches
R01 = Roty(-th1); %from frame 0 to frame 1
R10 = transpose(R01); %from 1 to Inertial
    
% Vertices
temp = [x,-0.025,0]+transpose(R10*[0;0;0.0125]);
Vertex1Data = GeoVerMakeBlock(temp, R10*Roty(-pi/2), [0.025,0.025,L]);
[X,Y,Z] = GeoPatMakeBlock(Vertex1Data);
    
Patch1Data_X = X;
Patch1Data_Y = Y;
Patch1Data_Z = Z;

%% Draw Motor1
% Calculate Rotation Matrix - from inertial to body
% Compute propagation of vertices and patches
%Vertices - may need to change the height
temp = [x,-0.025,0];
    
Vertex2Data = GeoVerMakeCyl( temp, Roty(th1), 0.03, 0.05 );
[X,Y,Z] = GeoPatMakeCyl(Vertex2Data);
    
Patch2Data_X = X;
Patch2Data_Y = Y;
Patch2Data_Z = Z;

%% Draw Link 2
% Calculate Rotation Matrix - from inertial to body
% Compute propagation of vertices and patches
R02 = Roty(-th1-th2);%from frame 0 to frame 2
R20 = transpose(R02); %from 2 to Inertial
    
% Vertices
temp = [x+(L*cos(th1)), -0.05, (L*sin(th1))]+transpose(R20*[0;0;0.0125]);
Vertex3Data = GeoVerMakeBlock(temp, R20*Roty(-pi/2), [0.025,0.025,L]);
[X,Y,Z] = GeoPatMakeBlock(Vertex3Data);
    
Patch3Data_X = X;
Patch3Data_Y = Y;
Patch3Data_Z = Z;

%% Draw Motor2
% Calculate Rotation Matrix - from inertial to body
% Compute propagation of vertices and patches

%Vertices - may need to change the height
temp = [x+(L*cos(th1)), 0, (L*sin(th1))]+[0,-0.05,0];
Vertex4Data = GeoVerMakeCyl( temp, Roty(th2), 0.03, 0.05 );
[X,Y,Z] = GeoPatMakeCyl(Vertex4Data);
    
Patch4Data_X = X;
Patch4Data_Y = Y;
Patch4Data_Z = Z;

%% Draw Box
% Calculate Rotation Matrix - from inertial to body
% Compute propagation of vertices and patches
R0b = Roty(-aBox);%from frame 0 to frame 2
Rb0 = transpose(R0b); %from 2 to Inertial   

% Vertices
temp = [xBox, -0.0875, zBox] + transpose(Rb0*[0;0;-0.05]);
Vertex6Data = GeoVerMakeBlock(temp, Rb0, [0.1,0.1,0.1]);
[X,Y,Z] = GeoPatMakeBlock(Vertex6Data);
    
Patch6Data_X = X;
Patch6Data_Y = Y;
Patch6Data_Z = Z;


    
%% PLOT
% Draw patches
persistent h0
persistent h1
persistent h2
persistent h3
persistent h4
persistent h5
persistent h6
persistent hground
persistent FigHandle
ground.vertices=[10 -10 -10; -10 -10 -10; -10 10 -10; 10 10 -10]*0.5; %square
ground.faces=[1 2 3 4]; %connect vertices

if isempty(FigHandle)
    close all;
    figure(1);
    FigHandle = gcf;
    h0 = patch(PatchData_X,PatchData_Y,PatchData_Z,'FaceColor','r');
    h5 = patch(Patch5Data_X,Patch5Data_Y,Patch5Data_Z,'FaceColor','c');
    h6 = patch(Patch6Data_X,Patch6Data_Y,Patch6Data_Z,'FaceColor','g');
    h1 = patch(Patch1Data_X,Patch1Data_Y,Patch1Data_Z,'FaceColor','r');
    h3 = patch(Patch3Data_X,Patch3Data_Y,Patch3Data_Z,'FaceColor','r');
    h2 = patch(Patch2Data_X,Patch2Data_Y,Patch2Data_Z,'FaceColor','r');
    h4 = patch(Patch4Data_X,Patch4Data_Y,Patch4Data_Z,'FaceColor','r');
    hground = patch('Faces',ground.faces,'Vertices',ground.vertices,'FaceColor',[211,211,211]/255);
end

set(hground,'FaceLighting','phong','EdgeLighting','phong','FaceAlpha',0.5);
hold on;

set(h0,'FaceLighting','phong','EdgeLighting','phong','FaceAlpha',1);
set(h5,'FaceLighting','phong','EdgeLighting','phong','FaceAlpha',1);
set(h6,'FaceLighting','phong','EdgeLighting','phong','FaceAlpha',1);
set(h1,'FaceLighting','phong','EdgeLighting','phong','FaceAlpha',1,'EdgeColor','k');
set(h2,'FaceLighting','phong','EdgeLighting','phong','FaceAlpha',1,'EdgeColor','k');
set(h3,'FaceLighting','phong','EdgeLighting','phong','FaceAlpha',1,'EdgeColor','k');
set(h4,'FaceLighting','phong','EdgeLighting','phong','FaceAlpha',1,'EdgeColor','k');
grid on

xlabel({'X Position (m)'},'FontSize',14,'FontName','AvantGarde');
ylabel({'Y Position (m)'},'FontSize',14,'FontName','AvantGarde');
zlabel({'Z Position (m)'},'FontSize',14,'FontName','AvantGarde');

% Create title
title({'2D Manipulator'},'FontWeight','bold','FontSize',24,...
    'FontName','AvantGarde');

axis([-0.6 0.6 -0.6 0.6 -0.6 0.6])
camlight;
grid on;
view([10,15]);
set(FigHandle, 'Position', [100, 100, 600, 400]);

set(h0,'XData',PatchData_X);
set(h0,'YData',PatchData_Y);
set(h0,'ZData',PatchData_Z);
set(h1,'XData',Patch1Data_X);
set(h1,'YData',Patch1Data_Y);
set(h1,'ZData',Patch1Data_Z);
set(h2,'XData',Patch2Data_X);
set(h2,'YData',Patch2Data_Y);
set(h2,'ZData',Patch2Data_Z);
set(h3,'XData',Patch3Data_X);
set(h3,'YData',Patch3Data_Y);
set(h3,'ZData',Patch3Data_Z);
set(h4,'XData',Patch4Data_X);
set(h4,'YData',Patch4Data_Y);
set(h4,'ZData',Patch4Data_Z);
set(h5,'XData',Patch5Data_X);
set(h5,'YData',Patch5Data_Y);
set(h5,'ZData',Patch5Data_Z);
set(h6,'XData',Patch6Data_X);
set(h6,'YData',Patch6Data_Y);
set(h6,'ZData',Patch6Data_Z);
drawnow;

xlim('manual')
ylim('manual')

end

%% Helper Functions

function A = Rotx(th)
    A = [1 0        0;...
         0 cos(th)  sin(th);...
         0 -sin(th)  cos(th)];
end

function A = Roty(th)
    A = [cos(th)  0   -sin(th);...
         0        1   0;...
         sin(th)  0   cos(th)];
end 

function A = Rotz(th)
    A = [cos(th)   sin(th) 0;... 
         -sin(th)  cos(th) 0;...
         0        0        1];
end

== matlab function LBSSHA005_EEE4119F_Project/Controller_no_box/G ==
  data: G output; th1 input; th2 input
function G = G(th1,th2)
%#codegen

%    This function was generated by the Symbolic Math Toolbox version 8.7.
%    13-May-2022 16:47:02

t2 = th1+th2;
t3 = cos(t2);
t4 = t3.*3.065625e-1;
G = [t4+cos(th1).*9.196875e-1,t4,0.0];

== matlab function LBSSHA005_EEE4119F_Project/Controller_no_box/J ==
  data: th1 input; J output; th2 input
function J = J(th1,th2)
%#codegen

%    This function was generated by the Symbolic Math Toolbox version 8.7.
%    13-May-2022 16:47:03

t2 = th1+th2;
t3 = cos(t2);
t4 = sin(t2);
t5 = t3./4.0;
t6 = t4./4.0;
t7 = -t6;
J = reshape([t7-sin(th1)./4.0,t5+cos(th1)./4.0,1.0,t7,t5,1.0,1.0,0.0,0.0],[3,3]);
